simulink model "corr_3ghz_lib"  (Simulink 6.2)
settings: Solver=ode45  StartTime=0.0  StopTime=10.0  RelTol=1e-3
undefined symbols (not defined in the file): cmult_4bit_em
libraries: xbsIndex_r3 x29, casper_library x21, xps_library x1
settings Model: LastModifiedBy=wjm
settings DebuggingCC: SolverPrmCheckMsg=warning

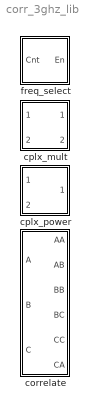
== system corr_3ghz_lib ==
  correlate : Subsystem
  cplx_mult : Subsystem
  cplx_power : Subsystem
  freq_select : Subsystem

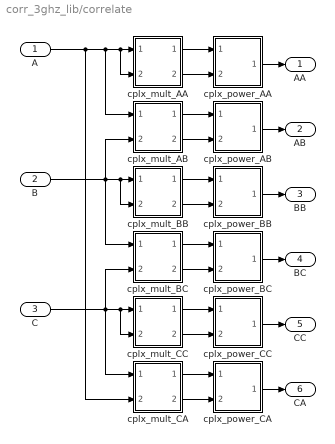
== system corr_3ghz_lib/correlate ==
  A : Inport  Port=1  LatchInput=off
  B : Inport  Port=2  LatchInput=off
  C : Inport  Port=3  LatchInput=off
  cplx_mult_AA : Subsystem
  cplx_mult_AB : Subsystem
  cplx_mult_BB : Subsystem
  cplx_mult_BC : Subsystem
  cplx_mult_CA : Subsystem
  cplx_mult_CC : Subsystem
  cplx_power_AA : Subsystem
  cplx_power_AB : Subsystem
  cplx_power_BB : Subsystem
  cplx_power_BC : Subsystem
  cplx_power_CA : Subsystem
  cplx_power_CC : Subsystem
  AA : Outport
  AB : Outport  Port=2
  BB : Outport  Port=3
  BC : Outport  Port=4
  CC : Outport  Port=5
  CA : Outport  Port=6
  wires:
  A/1 -> cplx_mult_AA/1(a+bi), cplx_mult_AA/2(c+di), cplx_mult_AB/1(a+bi), cplx_mult_CA/2(c+di)
  B/1 -> cplx_mult_BB/1(a+bi), cplx_mult_BB/2(c+di), cplx_mult_AB/2(c+di), cplx_mult_BC/1(a+bi)
  C/1 -> cplx_mult_CC/1(a+bi), cplx_mult_CC/2(c+di), cplx_mult_BC/2(c+di), cplx_mult_CA/1(a+bi)
  cplx_mult_AA/1(real) -> cplx_power_AA/1(real)
  cplx_mult_AA/2(imag) -> cplx_power_AA/2(imag)
  cplx_mult_AB/1(real) -> cplx_power_AB/1(real)
  cplx_mult_AB/2(imag) -> cplx_power_AB/2(imag)
  cplx_mult_BB/1(real) -> cplx_power_BB/1(real)
  cplx_mult_BB/2(imag) -> cplx_power_BB/2(imag)
  cplx_mult_BC/1(real) -> cplx_power_BC/1(real)
  cplx_mult_BC/2(imag) -> cplx_power_BC/2(imag)
  cplx_mult_CC/1(real) -> cplx_power_CC/1(real)
  cplx_mult_CC/2(imag) -> cplx_power_CC/2(imag)
  cplx_mult_CA/1(real) -> cplx_power_CA/1(real)
  cplx_mult_CA/2(imag) -> cplx_power_CA/2(imag)
  cplx_power_AA/1(pwr) -> AA/1
  cplx_power_AB/1(pwr) -> AB/1
  cplx_power_BB/1(pwr) -> BB/1
  cplx_power_BC/1(pwr) -> BC/1
  cplx_power_CC/1(pwr) -> CC/1
  cplx_power_CA/1(pwr) -> CA/1

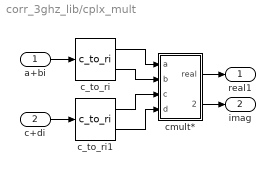
== system corr_3ghz_lib/cplx_mult ==
  a+bi : Inport  Port=1  LatchInput=off
  c+di : Inport  Port=2  LatchInput=off
  c_to_ri : casper_library/Misc/c_to_ri  n_bits=4  bin_pt=0
      settings: AttributesFormatString=4_0 r/i
  c_to_ri1 : casper_library/Misc/c_to_ri  n_bits=4  bin_pt=0
      settings: AttributesFormatString=4_0 r/i
  cmult* : Subsystem  BlockChoice=cmult_4bit_em*
      link override cmult_4bit_br*: mult_latency=mult_latency  add_latency=add_latency
      link override cmult_4bit_em*: mult_latency=mult_latency  add_latency=add_latency
      link override cmult_4bit_sl*: mult_latency=mult_latency  add_latency=add_latency
      settings: AttributesFormatString=%<BlockChoice>  TemplateBlock=casper_library/Multipliers/cmult*  MemberBlocks=cmult_4bit_br*,cmult_4bit_em*,cmult_4bit_sl*
      mask Type: cmult*
  real1 : Outport
  imag : Outport  Port=2
  wires:
  c_to_ri1/2 -> cmult*/4(d)
  c_to_ri1/1 -> cmult*/3(c)
  c+di/1 -> c_to_ri1/1
  c_to_ri/2 -> cmult*/2(b)
  c_to_ri/1 -> cmult*/1(a)
  a+bi/1 -> c_to_ri/1
  cmult*/1(real) -> real1/1
  cmult*/2(imag) -> imag/1

== system corr_3ghz_lib/cplx_power ==
  real : Inport  Port=1  LatchInput=off
  imag : Inport  Port=2  LatchInput=off
  imag_square : xbsIndex_r3/Mult  precision=Full  arith_type="Signed  (2's comp)"  n_bits=8  bin_pt=2  quantization=Truncate  overflow=Wrap  latency=4  explicit_period=on  period=1  en=off  dbl_ovrd=off  show_param=off  mult_type=Parallel  oversample=2  use_embedded=off  pipeline=on  use_rpm=on  placement_style=Rectangular Shape  gen_core=off
      settings: xl_area=[0, 0, 0, 0, 0, 0, 0]
  power_adder : xbsIndex_r3/AddSub  mode=Addition  precision=Full  arith_type=Unsigned  n_bits=8  bin_pt=2  quantization=Truncate  overflow=Wrap  latency=0  explicit_period=on  period=1  use_carryin=off  use_carryout=off  en=off  dbl_ovrd=off  show_param=off  use_core=on  pipeline=off  use_rpm=on  gen_core=off
      settings: xl_area=[0, 0, 0, 0, 0, 0, 0]
  real_square : xbsIndex_r3/Mult  precision=Full  arith_type="Signed  (2's comp)"  n_bits=8  bin_pt=2  quantization=Truncate  overflow=Wrap  latency=4  explicit_period=on  period=1  en=off  dbl_ovrd=off  show_param=off  mult_type=Parallel  oversample=2  use_embedded=off  pipeline=on  use_rpm=on  placement_style=Rectangular Shape  gen_core=off
      settings: xl_area=[0, 0, 0, 0, 0, 0, 0]
  pwr : Outport
  wires:
  real_square/1 -> power_adder/1
  imag_square/1 -> power_adder/2
  real/1 -> real_square/1, real_square/2
  imag/1 -> imag_square/2, imag_square/1
  power_adder/1 -> pwr/1

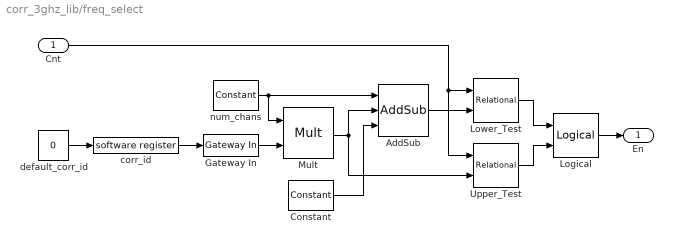
== system corr_3ghz_lib/freq_select ==
  Cnt : Inport  Port=1  LatchInput=off
  AddSub : xbsIndex_r3/AddSub  mode=Addition or Subtraction  precision=Full  arith_type=Unsigned  n_bits=8  bin_pt=2  quantization=Truncate  overflow=Wrap  latency=0  explicit_period=on  period=1  use_carryin=off  use_carryout=off  en=off  dbl_ovrd=off  show_param=off  use_core=on  pipeline=off  use_rpm=on  gen_core=off
      settings: xl_area=[0, 0, 0, 0, 0, 0, 0]
  Constant : xbsIndex_r3/Constant  const=1  equ=P=C  arith_type=Unsigned  n_bits=1  bin_pt=0  opselect=C  inp2=PCIN>>17  opr=+  inp1=P  carry=CIN  iostate=0  explicit_period=off  period=1  dbl_ovrd=off
  Gateway In : xbsIndex_r3/Gateway In  arith_type=Unsigned  n_bits=2  bin_pt=0  quantization=Truncate  overflow=Wrap  period=1  timing_constraint=None  locs_specified=off  LOCs={}  needs_fixed_name=off  dbl_ovrd=off  show_param=off
      settings: xl_area=[0, 0, 0, 0, 0, 0, 0]
  Logical : xbsIndex_r3/Logical  logical_function=AND  inputs=2  precision=Full  arith_type=Unsigned  n_bits=8  bin_pt=2  align_bp=on  latency=0  explicit_period=on  period=1  en=off  dbl_ovrd=off  show_param=off
      settings: xl_area=[0, 0, 0, 0, 0, 0, 0]
  Lower_Test : xbsIndex_r3/Relational  mode=a>b  latency=1  explicit_period=on  period=1  en=off  dbl_ovrd=off  show_param=off
      settings: xl_area=[0, 0, 0, 0, 0, 0, 0]
  Mult : xbsIndex_r3/Mult  precision=Full  arith_type="Signed  (2's comp)"  n_bits=8  bin_pt=2  quantization=Truncate  overflow=Wrap  latency=3  explicit_period=on  period=1  en=off  dbl_ovrd=off  show_param=off  mult_type=Parallel  oversample=2  use_embedded=off  pipeline=on  use_rpm=on  placement_style=Rectangular Shape  gen_core=off
      settings: xl_area=[0, 0, 0, 0, 0, 0, 0]
  Upper_Test : xbsIndex_r3/Relational  mode=a<b  latency=1  explicit_period=on  period=1  en=off  dbl_ovrd=off  show_param=off
      settings: xl_area=[0, 0, 0, 0, 0, 0, 0]
  corr_id : xps_library/software register  Tag=xps:sw_reg  io_dir=To Processor  arith_type=Unsigned  bitwidth=32  bin_pt=0  sample_period=1  gw_name=corr_3ghz_lib_freq_select_corr_id_user_data_in
  default_corr_id : Constant  Value=0  SampleTime=1
  num_chans : xbsIndex_r3/Constant  const=22  equ=P=C  arith_type=Unsigned  n_bits=5  bin_pt=0  opselect=C  inp2=PCIN>>17  opr=+  inp1=P  carry=CIN  iostate=0  explicit_period=on  period=1  dbl_ovrd=off
  En : Outport
  wires:
  Cnt/1 -> Lower_Test/1, Upper_Test/1
  Lower_Test/1 -> Logical/1
  Upper_Test/1 -> Logical/2
  default_corr_id/1 -> corr_id/1
  corr_id/1 -> Gateway In/1
  Gateway In/1 -> Mult/2
  Mult/1 -> AddSub/2, Upper_Test/2
  num_chans/1 -> AddSub/1, Mult/1
  Constant/1 -> AddSub/3
  AddSub/1 -> Lower_Test/2
  Logical/1 -> En/1

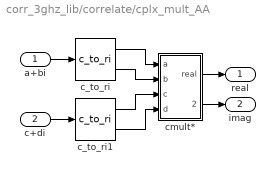
== system corr_3ghz_lib/correlate/cplx_mult_AA ==
  a+bi : Inport  Port=1  LatchInput=off
  c+di : Inport  Port=2  LatchInput=off
  c_to_ri : casper_library/Misc/c_to_ri  n_bits=4  bin_pt=0
      settings: AttributesFormatString=4_0 r/i
  c_to_ri1 : casper_library/Misc/c_to_ri  n_bits=4  bin_pt=0
      settings: AttributesFormatString=4_0 r/i
  cmult* : Subsystem  BlockChoice=cmult_4bit_em*
      link override cmult_4bit_br*: mult_latency=mult_latency  add_latency=add_latency
      link override cmult_4bit_em*: mult_latency=mult_latency  add_latency=add_latency
      link override cmult_4bit_sl*: mult_latency=mult_latency  add_latency=add_latency
      settings: AttributesFormatString=%<BlockChoice>  TemplateBlock=casper_library/Multipliers/cmult*  MemberBlocks=cmult_4bit_br*,cmult_4bit_em*,cmult_4bit_sl*
      mask Type: cmult*
  real : Outport
  imag : Outport  Port=2
  wires:
  c_to_ri1/2 -> cmult*/4(d)
  c_to_ri1/1 -> cmult*/3(c)
  c+di/1 -> c_to_ri1/1
  c_to_ri/2 -> cmult*/2(b)
  c_to_ri/1 -> cmult*/1(a)
  a+bi/1 -> c_to_ri/1
  cmult*/1(real) -> real/1
  cmult*/2(imag) -> imag/1

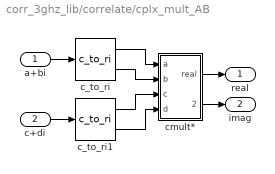
== system corr_3ghz_lib/correlate/cplx_mult_AB ==
  a+bi : Inport  Port=1  LatchInput=off
  c+di : Inport  Port=2  LatchInput=off
  c_to_ri : casper_library/Misc/c_to_ri  n_bits=4  bin_pt=0
      settings: AttributesFormatString=4_0 r/i
  c_to_ri1 : casper_library/Misc/c_to_ri  n_bits=4  bin_pt=0
      settings: AttributesFormatString=4_0 r/i
  cmult* : Subsystem  BlockChoice=cmult_4bit_em*
      link override cmult_4bit_br*: mult_latency=mult_latency  add_latency=add_latency
      link override cmult_4bit_em*: mult_latency=mult_latency  add_latency=add_latency
      link override cmult_4bit_sl*: mult_latency=mult_latency  add_latency=add_latency
      settings: AttributesFormatString=%<BlockChoice>  TemplateBlock=casper_library/Multipliers/cmult*  MemberBlocks=cmult_4bit_br*,cmult_4bit_em*,cmult_4bit_sl*
      mask Type: cmult*
  real : Outport
  imag : Outport  Port=2
  wires:
  c_to_ri1/2 -> cmult*/4(d)
  c_to_ri1/1 -> cmult*/3(c)
  c+di/1 -> c_to_ri1/1
  c_to_ri/2 -> cmult*/2(b)
  c_to_ri/1 -> cmult*/1(a)
  a+bi/1 -> c_to_ri/1
  cmult*/1(real) -> real/1
  cmult*/2(imag) -> imag/1

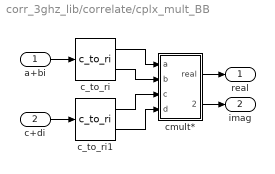
== system corr_3ghz_lib/correlate/cplx_mult_BB ==
  a+bi : Inport  Port=1  LatchInput=off
  c+di : Inport  Port=2  LatchInput=off
  c_to_ri : casper_library/Misc/c_to_ri  n_bits=4  bin_pt=0
      settings: AttributesFormatString=4_0 r/i
  c_to_ri1 : casper_library/Misc/c_to_ri  n_bits=4  bin_pt=0
      settings: AttributesFormatString=4_0 r/i
  cmult* : Subsystem  BlockChoice=cmult_4bit_em*
      link override cmult_4bit_br*: mult_latency=mult_latency  add_latency=add_latency
      link override cmult_4bit_em*: mult_latency=mult_latency  add_latency=add_latency
      link override cmult_4bit_sl*: mult_latency=mult_latency  add_latency=add_latency
      settings: AttributesFormatString=%<BlockChoice>  TemplateBlock=casper_library/Multipliers/cmult*  MemberBlocks=cmult_4bit_br*,cmult_4bit_em*,cmult_4bit_sl*
      mask Type: cmult*
  real : Outport
  imag : Outport  Port=2
  wires:
  c_to_ri1/2 -> cmult*/4(d)
  c_to_ri1/1 -> cmult*/3(c)
  c+di/1 -> c_to_ri1/1
  c_to_ri/2 -> cmult*/2(b)
  c_to_ri/1 -> cmult*/1(a)
  a+bi/1 -> c_to_ri/1
  cmult*/1(real) -> real/1
  cmult*/2(imag) -> imag/1

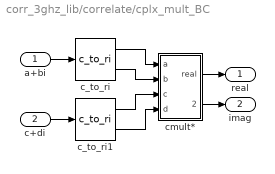
== system corr_3ghz_lib/correlate/cplx_mult_BC ==
  a+bi : Inport  Port=1  LatchInput=off
  c+di : Inport  Port=2  LatchInput=off
  c_to_ri : casper_library/Misc/c_to_ri  n_bits=4  bin_pt=0
      settings: AttributesFormatString=4_0 r/i
  c_to_ri1 : casper_library/Misc/c_to_ri  n_bits=4  bin_pt=0
      settings: AttributesFormatString=4_0 r/i
  cmult* : Subsystem  BlockChoice=cmult_4bit_em*
      link override cmult_4bit_br*: mult_latency=mult_latency  add_latency=add_latency
      link override cmult_4bit_em*: mult_latency=mult_latency  add_latency=add_latency
      link override cmult_4bit_sl*: mult_latency=mult_latency  add_latency=add_latency
      settings: AttributesFormatString=%<BlockChoice>  TemplateBlock=casper_library/Multipliers/cmult*  MemberBlocks=cmult_4bit_br*,cmult_4bit_em*,cmult_4bit_sl*
      mask Type: cmult*
  real : Outport
  imag : Outport  Port=2
  wires:
  c_to_ri1/2 -> cmult*/4(d)
  c_to_ri1/1 -> cmult*/3(c)
  c+di/1 -> c_to_ri1/1
  c_to_ri/2 -> cmult*/2(b)
  c_to_ri/1 -> cmult*/1(a)
  a+bi/1 -> c_to_ri/1
  cmult*/1(real) -> real/1
  cmult*/2(imag) -> imag/1

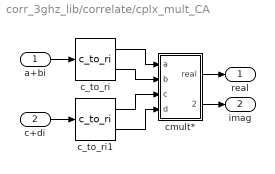
== system corr_3ghz_lib/correlate/cplx_mult_CA ==
  a+bi : Inport  Port=1  LatchInput=off
  c+di : Inport  Port=2  LatchInput=off
  c_to_ri : casper_library/Misc/c_to_ri  n_bits=4  bin_pt=0
      settings: AttributesFormatString=4_0 r/i
  c_to_ri1 : casper_library/Misc/c_to_ri  n_bits=4  bin_pt=0
      settings: AttributesFormatString=4_0 r/i
  cmult* : Subsystem  BlockChoice=cmult_4bit_em*
      link override cmult_4bit_br*: mult_latency=mult_latency  add_latency=add_latency
      link override cmult_4bit_em*: mult_latency=mult_latency  add_latency=add_latency
      link override cmult_4bit_sl*: mult_latency=mult_latency  add_latency=add_latency
      settings: AttributesFormatString=%<BlockChoice>  TemplateBlock=casper_library/Multipliers/cmult*  MemberBlocks=cmult_4bit_br*,cmult_4bit_em*,cmult_4bit_sl*
      mask Type: cmult*
  real : Outport
  imag : Outport  Port=2
  wires:
  c_to_ri1/2 -> cmult*/4(d)
  c_to_ri1/1 -> cmult*/3(c)
  c+di/1 -> c_to_ri1/1
  c_to_ri/2 -> cmult*/2(b)
  c_to_ri/1 -> cmult*/1(a)
  a+bi/1 -> c_to_ri/1
  cmult*/1(real) -> real/1
  cmult*/2(imag) -> imag/1

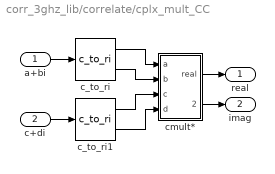
== system corr_3ghz_lib/correlate/cplx_mult_CC ==
  a+bi : Inport  Port=1  LatchInput=off
  c+di : Inport  Port=2  LatchInput=off
  c_to_ri : casper_library/Misc/c_to_ri  n_bits=4  bin_pt=0
      settings: AttributesFormatString=4_0 r/i
  c_to_ri1 : casper_library/Misc/c_to_ri  n_bits=4  bin_pt=0
      settings: AttributesFormatString=4_0 r/i
  cmult* : Subsystem  BlockChoice=cmult_4bit_em*
      link override cmult_4bit_br*: mult_latency=mult_latency  add_latency=add_latency
      link override cmult_4bit_em*: mult_latency=mult_latency  add_latency=add_latency
      link override cmult_4bit_sl*: mult_latency=mult_latency  add_latency=add_latency
      settings: AttributesFormatString=%<BlockChoice>  TemplateBlock=casper_library/Multipliers/cmult*  MemberBlocks=cmult_4bit_br*,cmult_4bit_em*,cmult_4bit_sl*
      mask Type: cmult*
  real : Outport
  imag : Outport  Port=2
  wires:
  c_to_ri1/2 -> cmult*/4(d)
  c_to_ri1/1 -> cmult*/3(c)
  c+di/1 -> c_to_ri1/1
  c_to_ri/2 -> cmult*/2(b)
  c_to_ri/1 -> cmult*/1(a)
  a+bi/1 -> c_to_ri/1
  cmult*/1(real) -> real/1
  cmult*/2(imag) -> imag/1

== system corr_3ghz_lib/correlate/cplx_power_AA ==
  real : Inport  Port=1  LatchInput=off
  imag : Inport  Port=2  LatchInput=off
  imag_square : xbsIndex_r3/Mult  precision=Full  arith_type="Signed  (2's comp)"  n_bits=8  bin_pt=2  quantization=Truncate  overflow=Wrap  latency=4  explicit_period=on  period=1  en=off  dbl_ovrd=off  show_param=off  mult_type=Parallel  oversample=2  use_embedded=off  pipeline=on  use_rpm=on  placement_style=Rectangular Shape  gen_core=off
      settings: xl_area=[0, 0, 0, 0, 0, 0, 0]
  power_adder : xbsIndex_r3/AddSub  mode=Addition  precision=Full  arith_type=Unsigned  n_bits=8  bin_pt=2  quantization=Truncate  overflow=Wrap  latency=0  explicit_period=on  period=1  use_carryin=off  use_carryout=off  en=off  dbl_ovrd=off  show_param=off  use_core=on  pipeline=off  use_rpm=on  gen_core=off
      settings: xl_area=[0, 0, 0, 0, 0, 0, 0]
  real_square : xbsIndex_r3/Mult  precision=Full  arith_type="Signed  (2's comp)"  n_bits=8  bin_pt=2  quantization=Truncate  overflow=Wrap  latency=4  explicit_period=on  period=1  en=off  dbl_ovrd=off  show_param=off  mult_type=Parallel  oversample=2  use_embedded=off  pipeline=on  use_rpm=on  placement_style=Rectangular Shape  gen_core=off
      settings: xl_area=[0, 0, 0, 0, 0, 0, 0]
  pwr : Outport
  wires:
  real_square/1 -> power_adder/1
  imag_square/1 -> power_adder/2
  real/1 -> real_square/1, real_square/2
  imag/1 -> imag_square/2, imag_square/1
  power_adder/1 -> pwr/1

== system corr_3ghz_lib/correlate/cplx_power_AB ==
  real : Inport  Port=1  LatchInput=off
  imag : Inport  Port=2  LatchInput=off
  imag_square : xbsIndex_r3/Mult  precision=Full  arith_type="Signed  (2's comp)"  n_bits=8  bin_pt=2  quantization=Truncate  overflow=Wrap  latency=4  explicit_period=on  period=1  en=off  dbl_ovrd=off  show_param=off  mult_type=Parallel  oversample=2  use_embedded=off  pipeline=on  use_rpm=on  placement_style=Rectangular Shape  gen_core=off
      settings: xl_area=[0, 0, 0, 0, 0, 0, 0]
  power_adder : xbsIndex_r3/AddSub  mode=Addition  precision=Full  arith_type=Unsigned  n_bits=8  bin_pt=2  quantization=Truncate  overflow=Wrap  latency=0  explicit_period=on  period=1  use_carryin=off  use_carryout=off  en=off  dbl_ovrd=off  show_param=off  use_core=on  pipeline=off  use_rpm=on  gen_core=off
      settings: xl_area=[0, 0, 0, 0, 0, 0, 0]
  real_square : xbsIndex_r3/Mult  precision=Full  arith_type="Signed  (2's comp)"  n_bits=8  bin_pt=2  quantization=Truncate  overflow=Wrap  latency=4  explicit_period=on  period=1  en=off  dbl_ovrd=off  show_param=off  mult_type=Parallel  oversample=2  use_embedded=off  pipeline=on  use_rpm=on  placement_style=Rectangular Shape  gen_core=off
      settings: xl_area=[0, 0, 0, 0, 0, 0, 0]
  pwr : Outport
  wires:
  real_square/1 -> power_adder/1
  imag_square/1 -> power_adder/2
  real/1 -> real_square/1, real_square/2
  imag/1 -> imag_square/2, imag_square/1
  power_adder/1 -> pwr/1

== system corr_3ghz_lib/correlate/cplx_power_BB ==
  real : Inport  Port=1  LatchInput=off
  imag : Inport  Port=2  LatchInput=off
  imag_square : xbsIndex_r3/Mult  precision=Full  arith_type="Signed  (2's comp)"  n_bits=8  bin_pt=2  quantization=Truncate  overflow=Wrap  latency=4  explicit_period=on  period=1  en=off  dbl_ovrd=off  show_param=off  mult_type=Parallel  oversample=2  use_embedded=off  pipeline=on  use_rpm=on  placement_style=Rectangular Shape  gen_core=off
      settings: xl_area=[0, 0, 0, 0, 0, 0, 0]
  power_adder : xbsIndex_r3/AddSub  mode=Addition  precision=Full  arith_type=Unsigned  n_bits=8  bin_pt=2  quantization=Truncate  overflow=Wrap  latency=0  explicit_period=on  period=1  use_carryin=off  use_carryout=off  en=off  dbl_ovrd=off  show_param=off  use_core=on  pipeline=off  use_rpm=on  gen_core=off
      settings: xl_area=[0, 0, 0, 0, 0, 0, 0]
  real_square : xbsIndex_r3/Mult  precision=Full  arith_type="Signed  (2's comp)"  n_bits=8  bin_pt=2  quantization=Truncate  overflow=Wrap  latency=4  explicit_period=on  period=1  en=off  dbl_ovrd=off  show_param=off  mult_type=Parallel  oversample=2  use_embedded=off  pipeline=on  use_rpm=on  placement_style=Rectangular Shape  gen_core=off
      settings: xl_area=[0, 0, 0, 0, 0, 0, 0]
  pwr : Outport
  wires:
  real_square/1 -> power_adder/1
  imag_square/1 -> power_adder/2
  real/1 -> real_square/1, real_square/2
  imag/1 -> imag_square/2, imag_square/1
  power_adder/1 -> pwr/1

== system corr_3ghz_lib/correlate/cplx_power_BC ==
  real : Inport  Port=1  LatchInput=off
  imag : Inport  Port=2  LatchInput=off
  imag_square : xbsIndex_r3/Mult  precision=Full  arith_type="Signed  (2's comp)"  n_bits=8  bin_pt=2  quantization=Truncate  overflow=Wrap  latency=4  explicit_period=on  period=1  en=off  dbl_ovrd=off  show_param=off  mult_type=Parallel  oversample=2  use_embedded=off  pipeline=on  use_rpm=on  placement_style=Rectangular Shape  gen_core=off
      settings: xl_area=[0, 0, 0, 0, 0, 0, 0]
  power_adder : xbsIndex_r3/AddSub  mode=Addition  precision=Full  arith_type=Unsigned  n_bits=8  bin_pt=2  quantization=Truncate  overflow=Wrap  latency=0  explicit_period=on  period=1  use_carryin=off  use_carryout=off  en=off  dbl_ovrd=off  show_param=off  use_core=on  pipeline=off  use_rpm=on  gen_core=off
      settings: xl_area=[0, 0, 0, 0, 0, 0, 0]
  real_square : xbsIndex_r3/Mult  precision=Full  arith_type="Signed  (2's comp)"  n_bits=8  bin_pt=2  quantization=Truncate  overflow=Wrap  latency=4  explicit_period=on  period=1  en=off  dbl_ovrd=off  show_param=off  mult_type=Parallel  oversample=2  use_embedded=off  pipeline=on  use_rpm=on  placement_style=Rectangular Shape  gen_core=off
      settings: xl_area=[0, 0, 0, 0, 0, 0, 0]
  pwr : Outport
  wires:
  real_square/1 -> power_adder/1
  imag_square/1 -> power_adder/2
  real/1 -> real_square/1, real_square/2
  imag/1 -> imag_square/2, imag_square/1
  power_adder/1 -> pwr/1

== system corr_3ghz_lib/correlate/cplx_power_CA ==
  real : Inport  Port=1  LatchInput=off
  imag : Inport  Port=2  LatchInput=off
  imag_square : xbsIndex_r3/Mult  precision=Full  arith_type="Signed  (2's comp)"  n_bits=8  bin_pt=2  quantization=Truncate  overflow=Wrap  latency=4  explicit_period=on  period=1  en=off  dbl_ovrd=off  show_param=off  mult_type=Parallel  oversample=2  use_embedded=off  pipeline=on  use_rpm=on  placement_style=Rectangular Shape  gen_core=off
      settings: xl_area=[0, 0, 0, 0, 0, 0, 0]
  power_adder : xbsIndex_r3/AddSub  mode=Addition  precision=Full  arith_type=Unsigned  n_bits=8  bin_pt=2  quantization=Truncate  overflow=Wrap  latency=0  explicit_period=on  period=1  use_carryin=off  use_carryout=off  en=off  dbl_ovrd=off  show_param=off  use_core=on  pipeline=off  use_rpm=on  gen_core=off
      settings: xl_area=[0, 0, 0, 0, 0, 0, 0]
  real_square : xbsIndex_r3/Mult  precision=Full  arith_type="Signed  (2's comp)"  n_bits=8  bin_pt=2  quantization=Truncate  overflow=Wrap  latency=4  explicit_period=on  period=1  en=off  dbl_ovrd=off  show_param=off  mult_type=Parallel  oversample=2  use_embedded=off  pipeline=on  use_rpm=on  placement_style=Rectangular Shape  gen_core=off
      settings: xl_area=[0, 0, 0, 0, 0, 0, 0]
  pwr : Outport
  wires:
  real_square/1 -> power_adder/1
  imag_square/1 -> power_adder/2
  real/1 -> real_square/1, real_square/2
  imag/1 -> imag_square/2, imag_square/1
  power_adder/1 -> pwr/1

== system corr_3ghz_lib/correlate/cplx_power_CC ==
  real : Inport  Port=1  LatchInput=off
  imag : Inport  Port=2  LatchInput=off
  imag_square : xbsIndex_r3/Mult  precision=Full  arith_type="Signed  (2's comp)"  n_bits=8  bin_pt=2  quantization=Truncate  overflow=Wrap  latency=4  explicit_period=on  period=1  en=off  dbl_ovrd=off  show_param=off  mult_type=Parallel  oversample=2  use_embedded=off  pipeline=on  use_rpm=on  placement_style=Rectangular Shape  gen_core=off
      settings: xl_area=[0, 0, 0, 0, 0, 0, 0]
  power_adder : xbsIndex_r3/AddSub  mode=Addition  precision=Full  arith_type=Unsigned  n_bits=8  bin_pt=2  quantization=Truncate  overflow=Wrap  latency=0  explicit_period=on  period=1  use_carryin=off  use_carryout=off  en=off  dbl_ovrd=off  show_param=off  use_core=on  pipeline=off  use_rpm=on  gen_core=off
      settings: xl_area=[0, 0, 0, 0, 0, 0, 0]
  real_square : xbsIndex_r3/Mult  precision=Full  arith_type="Signed  (2's comp)"  n_bits=8  bin_pt=2  quantization=Truncate  overflow=Wrap  latency=4  explicit_period=on  period=1  en=off  dbl_ovrd=off  show_param=off  mult_type=Parallel  oversample=2  use_embedded=off  pipeline=on  use_rpm=on  placement_style=Rectangular Shape  gen_core=off
      settings: xl_area=[0, 0, 0, 0, 0, 0, 0]
  pwr : Outport
  wires:
  real_square/1 -> power_adder/1
  imag_square/1 -> power_adder/2
  real/1 -> real_square/1, real_square/2
  imag/1 -> imag_square/2, imag_square/1
  power_adder/1 -> pwr/1

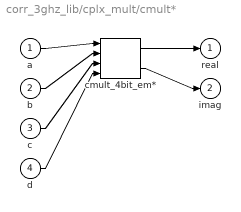
== system corr_3ghz_lib/cplx_mult/cmult* ==
  a : Inport  Port=1  LatchInput=off
  b : Inport  Port=2  LatchInput=off
  c : Inport  Port=3  LatchInput=off
  d : Inport  Port=4  LatchInput=off
  cmult_4bit_em* : casper_library/Multipliers/cmult_4bit_em*  mult_latency=mult_latency  add_latency=add_latency
  real : Outport
  imag : Outport  Port=2
  wires:
  a/1 -> cmult_4bit_em*/1
  b/1 -> cmult_4bit_em*/2
  c/1 -> cmult_4bit_em*/3
  d/1 -> cmult_4bit_em*/4
  cmult_4bit_em*/1 -> real/1
  cmult_4bit_em*/2 -> imag/1

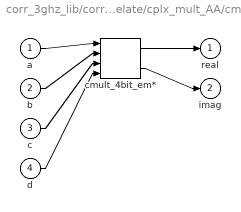
== system corr_3ghz_lib/correlate/cplx_mult_AA/cmult* ==
  a : Inport  Port=1  LatchInput=off
  b : Inport  Port=2  LatchInput=off
  c : Inport  Port=3  LatchInput=off
  d : Inport  Port=4  LatchInput=off
  cmult_4bit_em* : casper_library/Multipliers/cmult_4bit_em*  mult_latency=mult_latency  add_latency=add_latency
  real : Outport
  imag : Outport  Port=2
  wires:
  a/1 -> cmult_4bit_em*/1
  b/1 -> cmult_4bit_em*/2
  c/1 -> cmult_4bit_em*/3
  d/1 -> cmult_4bit_em*/4
  cmult_4bit_em*/1 -> real/1
  cmult_4bit_em*/2 -> imag/1

== system corr_3ghz_lib/correlate/cplx_mult_AB/cmult* ==
  a : Inport  Port=1  LatchInput=off
  b : Inport  Port=2  LatchInput=off
  c : Inport  Port=3  LatchInput=off
  d : Inport  Port=4  LatchInput=off
  cmult_4bit_em* : casper_library/Multipliers/cmult_4bit_em*  mult_latency=mult_latency  add_latency=add_latency
  real : Outport
  imag : Outport  Port=2
  wires:
  a/1 -> cmult_4bit_em*/1
  b/1 -> cmult_4bit_em*/2
  c/1 -> cmult_4bit_em*/3
  d/1 -> cmult_4bit_em*/4
  cmult_4bit_em*/1 -> real/1
  cmult_4bit_em*/2 -> imag/1

== system corr_3ghz_lib/correlate/cplx_mult_BB/cmult* ==
  a : Inport  Port=1  LatchInput=off
  b : Inport  Port=2  LatchInput=off
  c : Inport  Port=3  LatchInput=off
  d : Inport  Port=4  LatchInput=off
  cmult_4bit_em* : casper_library/Multipliers/cmult_4bit_em*  mult_latency=mult_latency  add_latency=add_latency
  real : Outport
  imag : Outport  Port=2
  wires:
  a/1 -> cmult_4bit_em*/1
  b/1 -> cmult_4bit_em*/2
  c/1 -> cmult_4bit_em*/3
  d/1 -> cmult_4bit_em*/4
  cmult_4bit_em*/1 -> real/1
  cmult_4bit_em*/2 -> imag/1

== system corr_3ghz_lib/correlate/cplx_mult_BC/cmult* ==
  a : Inport  Port=1  LatchInput=off
  b : Inport  Port=2  LatchInput=off
  c : Inport  Port=3  LatchInput=off
  d : Inport  Port=4  LatchInput=off
  cmult_4bit_em* : casper_library/Multipliers/cmult_4bit_em*  mult_latency=mult_latency  add_latency=add_latency
  real : Outport
  imag : Outport  Port=2
  wires:
  a/1 -> cmult_4bit_em*/1
  b/1 -> cmult_4bit_em*/2
  c/1 -> cmult_4bit_em*/3
  d/1 -> cmult_4bit_em*/4
  cmult_4bit_em*/1 -> real/1
  cmult_4bit_em*/2 -> imag/1

== system corr_3ghz_lib/correlate/cplx_mult_CA/cmult* ==
  a : Inport  Port=1  LatchInput=off
  b : Inport  Port=2  LatchInput=off
  c : Inport  Port=3  LatchInput=off
  d : Inport  Port=4  LatchInput=off
  cmult_4bit_em* : casper_library/Multipliers/cmult_4bit_em*  mult_latency=mult_latency  add_latency=add_latency
  real : Outport
  imag : Outport  Port=2
  wires:
  a/1 -> cmult_4bit_em*/1
  b/1 -> cmult_4bit_em*/2
  c/1 -> cmult_4bit_em*/3
  d/1 -> cmult_4bit_em*/4
  cmult_4bit_em*/1 -> real/1
  cmult_4bit_em*/2 -> imag/1

== system corr_3ghz_lib/correlate/cplx_mult_CC/cmult* ==
  a : Inport  Port=1  LatchInput=off
  b : Inport  Port=2  LatchInput=off
  c : Inport  Port=3  LatchInput=off
  d : Inport  Port=4  LatchInput=off
  cmult_4bit_em* : casper_library/Multipliers/cmult_4bit_em*  mult_latency=mult_latency  add_latency=add_latency
  real : Outport
  imag : Outport  Port=2
  wires:
  a/1 -> cmult_4bit_em*/1
  b/1 -> cmult_4bit_em*/2
  c/1 -> cmult_4bit_em*/3
  d/1 -> cmult_4bit_em*/4
  cmult_4bit_em*/1 -> real/1
  cmult_4bit_em*/2 -> imag/1
